simulink model "MSBR_Plant"  (R2021b)
settings: Solver=ode45  StartTime=0.0  StopTime=sim_time  MaxStep=ts_max  RelTol=1e-4
values from neighbouring files (symbols this model uses):
  a_1 = 8.7292e-2/wilson_ratio    (= 0.0087292)    [Whole_Plant_Cool_Pump_Accident_script.m]    (also in Whole_Plant_Fert_Pump_Accident_script.m; Whole_Plant_Fuel_Pump_Accident.m; Whole_Plant_Fuel_Pump_Accident_script.m; Whole_Plant_Reactivity_Accident.m)
  a_2 = 7.3787e-4/wilson_ratio    (= 7.3787e-05)    [Whole_Plant_Cool_Pump_Accident_script.m]    (also in Whole_Plant_Fert_Pump_Accident_script.m; Whole_Plant_Fuel_Pump_Accident.m; Whole_Plant_Fuel_Pump_Accident_script.m; Whole_Plant_Reactivity_Accident.m)
  a_b = 1.656e-5    (= 1.656e-05)    [Whole_Plant_Cool_Pump_Accident_script.m]    (also in Whole_Plant_Fert_Pump_Accident_script.m; Whole_Plant_Fuel_Pump_Accident.m; Whole_Plant_Fuel_Pump_Accident_script.m; Whole_Plant_Reactivity_Accident.m)
  a_f = -8.172e-5    (= -8.172e-05)    [Whole_Plant_Cool_Pump_Accident_script.m]    (also in Whole_Plant_Fert_Pump_Accident_script.m; Whole_Plant_Fuel_Pump_Accident.m; Whole_Plant_Fuel_Pump_Accident_script.m; Whole_Plant_Reactivity_Accident.m)
  a_g = 2.016e-5    (= 2.016e-05)    [Whole_Plant_Cool_Pump_Accident_script.m]    (also in Whole_Plant_Fert_Pump_Accident_script.m; Whole_Plant_Fuel_Pump_Accident.m; Whole_Plant_Fuel_Pump_Accident_script.m; Whole_Plant_Reactivity_Accident.m)
  A_s = pi()*((D_OTSG_i^2)/4) - A_w_OTSG - A_p_OTSG    [Whole_Plant_Cool_Pump_Accident_script.m]    (also in Whole_Plant_Fert_Pump_Accident_script.m; Whole_Plant_Fuel_Pump_Accident.m; Whole_Plant_Fuel_Pump_Accident_script.m; Whole_Plant_Reactivity_Accident.m)
  alpha_co = 316.2    [Whole_Plant_Cool_Pump_Accident_script.m]    (also in Whole_Plant_Fert_Pump_Accident_script.m; Whole_Plant_Fuel_Pump_Accident.m; Whole_Plant_Fuel_Pump_Accident_script.m; Whole_Plant_Reactivity_Accident.m)
  beta = [2.290e-04, 8.320e-04, 7.100e-04, 8.520e-04, 1.710e-04, 1.020e-04]    [Whole_Plant_Cool_Pump_Accident_script.m]    (also in Whole_Plant_Fert_Pump_Accident_script.m; Whole_Plant_Fuel_Pump_Accident.m; Whole_Plant_Fuel_Pump_Accident_script.m; Whole_Plant_Reactivity_Accident.m)
  beta_co = 68.0958    [Whole_Plant_Cool_Pump_Accident_script.m]    (also in Whole_Plant_Fert_Pump_Accident_script.m; Whole_Plant_Fuel_Pump_Accident.m; Whole_Plant_Fuel_Pump_Accident_script.m; Whole_Plant_Reactivity_Accident.m)
  beta_t = sum(beta)    [Whole_Plant_Cool_Pump_Accident_script.m]    (also in Whole_Plant_Fert_Pump_Accident_script.m; Whole_Plant_Fuel_Pump_Accident.m; Whole_Plant_Fuel_Pump_Accident_script.m; Whole_Plant_Reactivity_Accident.m)
  C_nc_X_A_nc = 12.8    [Whole_Plant_Cool_Pump_Accident_script.m]    (also in Whole_Plant_Fert_Pump_Accident_script.m; Whole_Plant_Fuel_Pump_Accident.m; Whole_Plant_Fuel_Pump_Accident_script.m; Whole_Plant_Reactivity_Accident.m)
  C_pcw = 0.0042    [Whole_Plant_Cool_Pump_Accident_script.m]    (also in Whole_Plant_Fert_Pump_Accident_script.m; Whole_Plant_Fuel_Pump_Accident.m; Whole_Plant_Fuel_Pump_Accident_script.m; Whole_Plant_Reactivity_Accident.m)
  C_rh_X_A_rh = 33    [Whole_Plant_Cool_Pump_Accident_script.m]    (also in Whole_Plant_Fert_Pump_Accident_script.m; Whole_Plant_Fuel_Pump_Accident.m; Whole_Plant_Fuel_Pump_Accident_script.m; Whole_Plant_Reactivity_Accident.m)
  C_v = 0.84    [Whole_Plant_Cool_Pump_Accident_script.m]    (also in Whole_Plant_Fert_Pump_Accident_script.m; Whole_Plant_Fuel_Pump_Accident.m; Whole_Plant_Fuel_Pump_Accident_script.m; Whole_Plant_Reactivity_Accident.m)
  ce1 = 1.2471e-07    [Whole_Plant_Cool_Pump_Accident_script.m]    (also in Whole_Plant_Fert_Pump_Accident_script.m; Whole_Plant_Fuel_Pump_Accident.m; Whole_Plant_Fuel_Pump_Accident_script.m; Whole_Plant_Reactivity_Accident.m)
  ce2 = 5.3816e-14    [Whole_Plant_Cool_Pump_Accident_script.m]    (also in Whole_Plant_Fert_Pump_Accident_script.m; Whole_Plant_Fuel_Pump_Accident.m; Whole_Plant_Fuel_Pump_Accident_script.m; Whole_Plant_Reactivity_Accident.m)
  ce3 = 3.3721e-08    [Whole_Plant_Cool_Pump_Accident_script.m]    (also in Whole_Plant_Fert_Pump_Accident_script.m; Whole_Plant_Fuel_Pump_Accident.m; Whole_Plant_Fuel_Pump_Accident_script.m; Whole_Plant_Reactivity_Accident.m)
  Cp_fw = XSteam('Cp_pT',P_set*10,T_fw)/1000    [Whole_Plant_Cool_Pump_Accident_script.m]    (also in Whole_Plant_Fert_Pump_Accident_script.m; Whole_Plant_Fuel_Pump_Accident.m; Whole_Plant_Fuel_Pump_Accident_script.m; Whole_Plant_Reactivity_Accident.m)
  Cp_p = Cp_sec    (= 0.001716588)    [Whole_Plant_Cool_Pump_Accident_script.m]    (also in Whole_Plant_Fert_Pump_Accident_script.m; Whole_Plant_Fuel_Pump_Accident.m; Whole_Plant_Fuel_Pump_Accident_script.m; Whole_Plant_Reactivity_Accident.m)
  Cp_rh = 0.0021520    (= 0.002152)    [Whole_Plant_Cool_Pump_Accident_script.m]    (also in Whole_Plant_Fert_Pump_Accident_script.m; Whole_Plant_Fuel_Pump_Accident.m; Whole_Plant_Fuel_Pump_Accident_script.m; Whole_Plant_Reactivity_Accident.m)
  Cp_s = XSteam('Cp_pT',P_s*10,T_s)/1000    [Whole_Plant_Cool_Pump_Accident_script.m]    (also in Whole_Plant_Fert_Pump_Accident_script.m; Whole_Plant_Fuel_Pump_Accident.m; Whole_Plant_Fuel_Pump_Accident_script.m; Whole_Plant_Reactivity_Accident.m)
  Cp_sc = XSteam('Cp_pT',P_set*10,T_sc2)/1000    [Whole_Plant_Cool_Pump_Accident_script.m]    (also in Whole_Plant_Fert_Pump_Accident_script.m; Whole_Plant_Fuel_Pump_Accident.m; Whole_Plant_Fuel_Pump_Accident_script.m; Whole_Plant_Reactivity_Accident.m)
  Cp_w = 468.992e-6    (= 0.000468992)    [Whole_Plant_Cool_Pump_Accident_script.m]    (also in Whole_Plant_Fert_Pump_Accident_script.m; Whole_Plant_Fuel_Pump_Accident.m; Whole_Plant_Fuel_Pump_Accident_script.m; Whole_Plant_Reactivity_Accident.m)
  D_it = D_ot-2*T_th    (= 0.014147)    [Whole_Plant_Cool_Pump_Accident_script.m]    (also in Whole_Plant_Fert_Pump_Accident_script.m; Whole_Plant_Fuel_Pump_Accident.m; Whole_Plant_Fuel_Pump_Accident_script.m; Whole_Plant_Reactivity_Accident.m)
  D_ot = 0.015875    [Whole_Plant_Cool_Pump_Accident_script.m]    (also in Whole_Plant_Fert_Pump_Accident_script.m; Whole_Plant_Fuel_Pump_Accident.m; Whole_Plant_Fuel_Pump_Accident_script.m; Whole_Plant_Reactivity_Accident.m)
  dHs_dPs = c(1)    [Whole_Plant_Cool_Pump_Accident_script.m]    (also in Whole_Plant_Fert_Pump_Accident_script.m; Whole_Plant_Fuel_Pump_Accident.m; Whole_Plant_Fuel_Pump_Accident_script.m; Whole_Plant_Reactivity_Accident.m)
  eta_hp_isen = 0.861    [Whole_Plant_Cool_Pump_Accident_script.m]    (also in Whole_Plant_Fert_Pump_Accident_script.m; Whole_Plant_Fuel_Pump_Accident.m; Whole_Plant_Fuel_Pump_Accident_script.m; Whole_Plant_Reactivity_Accident.m)
  eta_lp_isen = 0.861    [Whole_Plant_Cool_Pump_Accident_script.m]    (also in Whole_Plant_Fert_Pump_Accident_script.m; Whole_Plant_Fuel_Pump_Accident.m; Whole_Plant_Fuel_Pump_Accident_script.m; Whole_Plant_Reactivity_Accident.m)
  gamma_I = 5.1135e-2    (= 0.051135)    [Whole_Plant_Cool_Pump_Accident_script.m]    (also in Whole_Plant_Fert_Pump_Accident_script.m; Whole_Plant_Fuel_Pump_Accident.m; Whole_Plant_Fuel_Pump_Accident_script.m; Whole_Plant_Reactivity_Accident.m)
  gamma_Xe = 1.1628e-2    (= 0.011628)    [Whole_Plant_Cool_Pump_Accident_script.m]    (also in Whole_Plant_Fert_Pump_Accident_script.m; Whole_Plant_Fuel_Pump_Accident.m; Whole_Plant_Fuel_Pump_Accident_script.m; Whole_Plant_Reactivity_Accident.m)
  H_co0 = 0.149    [Whole_Plant_Cool_Pump_Accident_script.m]    (also in Whole_Plant_Fert_Pump_Accident_script.m; Whole_Plant_Fuel_Pump_Accident.m; Whole_Plant_Fuel_Pump_Accident_script.m; Whole_Plant_Reactivity_Accident.m)
  H_f_co0 = 0.149    [Whole_Plant_Cool_Pump_Accident_script.m]    (also in Whole_Plant_Fert_Pump_Accident_script.m; Whole_Plant_Fuel_Pump_Accident.m; Whole_Plant_Fuel_Pump_Accident_script.m; Whole_Plant_Reactivity_Accident.m)
  H_fg_co0 = 2.35    [Whole_Plant_Cool_Pump_Accident_script.m]    (also in Whole_Plant_Fert_Pump_Accident_script.m; Whole_Plant_Fuel_Pump_Accident.m; Whole_Plant_Fuel_Pump_Accident_script.m; Whole_Plant_Reactivity_Accident.m)
  H_fgrh0 = (XSteam('hV_p', P_s*1e1) - XSteam('hL_p', P_s*1e1))/1e3    [Whole_Plant_Cool_Pump_Accident_script.m]    (also in Whole_Plant_Fert_Pump_Accident_script.m; Whole_Plant_Fuel_Pump_Accident.m; Whole_Plant_Fuel_Pump_Accident_script.m; Whole_Plant_Reactivity_Accident.m)
  H_frh0 = XSteam('hL_p', P_s*1e1)/1e3    [Whole_Plant_Cool_Pump_Accident_script.m]    (also in Whole_Plant_Fert_Pump_Accident_script.m; Whole_Plant_Fuel_Pump_Accident.m; Whole_Plant_Fuel_Pump_Accident_script.m; Whole_Plant_Reactivity_Accident.m)
  h_fwh1 = 0.5927    [Whole_Plant_Cool_Pump_Accident_script.m]    (also in Whole_Plant_Fert_Pump_Accident_script.m; Whole_Plant_Fuel_Pump_Accident.m; Whole_Plant_Fuel_Pump_Accident_script.m; Whole_Plant_Reactivity_Accident.m)
  H_fwh10 = 0.46009    [Whole_Plant_Cool_Pump_Accident_script.m]    (also in Whole_Plant_Fert_Pump_Accident_script.m; Whole_Plant_Fuel_Pump_Accident.m; Whole_Plant_Fuel_Pump_Accident_script.m; Whole_Plant_Reactivity_Accident.m)
  h_fwh2 = 1.230803    [Whole_Plant_Cool_Pump_Accident_script.m]    (also in Whole_Plant_Fert_Pump_Accident_script.m; Whole_Plant_Fuel_Pump_Accident.m; Whole_Plant_Fuel_Pump_Accident_script.m; Whole_Plant_Reactivity_Accident.m)
  H_fwh20 = 0.6784    [Whole_Plant_Cool_Pump_Accident_script.m]    (also in Whole_Plant_Fert_Pump_Accident_script.m; Whole_Plant_Fuel_Pump_Accident.m; Whole_Plant_Fuel_Pump_Accident_script.m; Whole_Plant_Reactivity_Accident.m)
  H_grh0 = 2.8029    [Whole_Plant_Cool_Pump_Accident_script.m]    (also in Whole_Plant_Fert_Pump_Accident_script.m; Whole_Plant_Fuel_Pump_Accident.m; Whole_Plant_Fuel_Pump_Accident_script.m; Whole_Plant_Reactivity_Accident.m)
  H_hp_isen0 = 2.5111    [Whole_Plant_Cool_Pump_Accident_script.m]    (also in Whole_Plant_Fert_Pump_Accident_script.m; Whole_Plant_Fuel_Pump_Accident.m; Whole_Plant_Fuel_Pump_Accident_script.m; Whole_Plant_Reactivity_Accident.m)
  H_hpt_out = 2.6201    [Whole_Plant_Cool_Pump_Accident_script.m]    (also in Whole_Plant_Fert_Pump_Accident_script.m; Whole_Plant_Fuel_Pump_Accident.m; Whole_Plant_Fuel_Pump_Accident_script.m; Whole_Plant_Reactivity_Accident.m)
  H_lp_isen = 958.4*1054.35e-6/0.45359237    (= 2.22774699671)    [Whole_Plant_Cool_Pump_Accident_script.m]    (also in Whole_Plant_Fert_Pump_Accident_script.m; Whole_Plant_Fuel_Pump_Accident.m; Whole_Plant_Fuel_Pump_Accident_script.m; Whole_Plant_Reactivity_Accident.m)
  H_lpt_out = 2.3089    [Whole_Plant_Cool_Pump_Accident_script.m]    (also in Whole_Plant_Fert_Pump_Accident_script.m; Whole_Plant_Fuel_Pump_Accident.m; Whole_Plant_Fuel_Pump_Accident_script.m; Whole_Plant_Reactivity_Accident.m)
  H_nc = XSteam('h_pT', P_s*10, T_s)/1000    [Whole_Plant_Cool_Pump_Accident_script.m]    (also in Whole_Plant_Fert_Pump_Accident_script.m; Whole_Plant_Fuel_Pump_Accident.m; Whole_Plant_Fuel_Pump_Accident_script.m; Whole_Plant_Reactivity_Accident.m)
  h_pw = h_s    (= 0.02555)    [Whole_Plant_Cool_Pump_Accident_script.m]    (also in Whole_Plant_Fert_Pump_Accident_script.m; Whole_Plant_Fuel_Pump_Accident.m; Whole_Plant_Fuel_Pump_Accident_script.m; Whole_Plant_Reactivity_Accident.m)
  H_rh = 2.8115    [Whole_Plant_Cool_Pump_Accident_script.m]    (also in Whole_Plant_Fert_Pump_Accident_script.m; Whole_Plant_Fuel_Pump_Accident.m; Whole_Plant_Fuel_Pump_Accident_script.m; Whole_Plant_Reactivity_Accident.m)
  h_wb = 13349.334646671E-6    (= 0.0133493346467)    [Whole_Plant_Cool_Pump_Accident_script.m]    (also in Whole_Plant_Fert_Pump_Accident_script.m; Whole_Plant_Fuel_Pump_Accident.m; Whole_Plant_Fuel_Pump_Accident_script.m; Whole_Plant_Reactivity_Accident.m)
  h_ws = 5732.378387768E-6    (= 0.00573237838777)    [Whole_Plant_Cool_Pump_Accident_script.m]    (also in Whole_Plant_Fert_Pump_Accident_script.m; Whole_Plant_Fuel_Pump_Accident.m; Whole_Plant_Fuel_Pump_Accident_script.m; Whole_Plant_Reactivity_Accident.m)
  h_wsc = 8385.005556375E-6    (= 0.00838500555638)    [Whole_Plant_Cool_Pump_Accident_script.m]    (also in Whole_Plant_Fert_Pump_Accident_script.m; Whole_Plant_Fuel_Pump_Accident.m; Whole_Plant_Fuel_Pump_Accident_script.m; Whole_Plant_Reactivity_Accident.m)
  hA_bg = A_fert*h_bg    (= 2.76411813627)    [Whole_Plant_Cool_Pump_Accident_script.m]    (also in Whole_Plant_Fert_Pump_Accident_script.m; Whole_Plant_Fuel_Pump_Accident.m; Whole_Plant_Fuel_Pump_Accident_script.m; Whole_Plant_Reactivity_Accident.m)
  hA_co0 = 140    [Whole_Plant_Cool_Pump_Accident_script.m]    (also in Whole_Plant_Fert_Pump_Accident_script.m; Whole_Plant_Fuel_Pump_Accident.m; Whole_Plant_Fuel_Pump_Accident_script.m; Whole_Plant_Reactivity_Accident.m)
  hA_fg_dn = h_fg*A_fuel_down    [Whole_Plant_Cool_Pump_Accident_script.m]    (also in Whole_Plant_Fert_Pump_Accident_script.m; Whole_Plant_Fuel_Pump_Accident.m; Whole_Plant_Fuel_Pump_Accident_script.m; Whole_Plant_Reactivity_Accident.m)
  hA_fg_up = h_fg*A_fuel_up    [Whole_Plant_Cool_Pump_Accident_script.m]    (also in Whole_Plant_Fert_Pump_Accident_script.m; Whole_Plant_Fuel_Pump_Accident.m; Whole_Plant_Fuel_Pump_Accident_script.m; Whole_Plant_Reactivity_Accident.m)
  hA_p_bhx1 = [h_pb*A_pbhx/2,h_pb*A_pbhx/2]    [Whole_Plant_Cool_Pump_Accident_script.m]    (also in Whole_Plant_Fert_Pump_Accident_script.m; Whole_Plant_Fuel_Pump_Accident.m; Whole_Plant_Fuel_Pump_Accident_script.m; Whole_Plant_Reactivity_Accident.m)
  hA_p_bhx2 = hA_p_bhx1    [Whole_Plant_Cool_Pump_Accident_script.m]    (also in Whole_Plant_Fert_Pump_Accident_script.m; Whole_Plant_Fuel_Pump_Accident.m; Whole_Plant_Fuel_Pump_Accident_script.m; Whole_Plant_Reactivity_Accident.m)
  hA_p_bhx3 = hA_p_bhx1    [Whole_Plant_Cool_Pump_Accident_script.m]    (also in Whole_Plant_Fert_Pump_Accident_script.m; Whole_Plant_Fuel_Pump_Accident.m; Whole_Plant_Fuel_Pump_Accident_script.m; Whole_Plant_Reactivity_Accident.m)
  hA_p_bhx4 = hA_p_bhx1    [Whole_Plant_Cool_Pump_Accident_script.m]    (also in Whole_Plant_Fert_Pump_Accident_script.m; Whole_Plant_Fuel_Pump_Accident.m; Whole_Plant_Fuel_Pump_Accident_script.m; Whole_Plant_Reactivity_Accident.m)
  hA_p_fhx1 = [h_p*A_pfhx_dn/2,h_p*A_pfhx_dn/2,h_p*A_pfhx_up/2,h_p*A_pfhx_up/2]    [Whole_Plant_Cool_Pump_Accident_script.m]    (also in Whole_Plant_Fert_Pump_Accident_script.m; Whole_Plant_Fuel_Pump_Accident.m; Whole_Plant_Fuel_Pump_Accident_script.m; Whole_Plant_Reactivity_Accident.m)
  hA_p_fhx2 = hA_p_fhx1    [Whole_Plant_Cool_Pump_Accident_script.m]    (also in Whole_Plant_Fert_Pump_Accident_script.m; Whole_Plant_Fuel_Pump_Accident.m; Whole_Plant_Fuel_Pump_Accident_script.m; Whole_Plant_Reactivity_Accident.m)
  hA_p_fhx3 = hA_p_fhx1    [Whole_Plant_Cool_Pump_Accident_script.m]    (also in Whole_Plant_Fert_Pump_Accident_script.m; Whole_Plant_Fuel_Pump_Accident.m; Whole_Plant_Fuel_Pump_Accident_script.m; Whole_Plant_Reactivity_Accident.m)
  hA_p_fhx4 = hA_p_fhx1    [Whole_Plant_Cool_Pump_Accident_script.m]    (also in Whole_Plant_Fert_Pump_Accident_script.m; Whole_Plant_Fuel_Pump_Accident.m; Whole_Plant_Fuel_Pump_Accident_script.m; Whole_Plant_Reactivity_Accident.m)
  hA_s_bhx1 = [h_sb*A_sbhx/2,h_sb*A_sbhx/2]    [Whole_Plant_Cool_Pump_Accident_script.m]    (also in Whole_Plant_Fert_Pump_Accident_script.m; Whole_Plant_Fuel_Pump_Accident.m; Whole_Plant_Fuel_Pump_Accident_script.m; Whole_Plant_Reactivity_Accident.m)
  hA_s_bhx2 = hA_s_bhx1    [Whole_Plant_Cool_Pump_Accident_script.m]    (also in Whole_Plant_Fert_Pump_Accident_script.m; Whole_Plant_Fuel_Pump_Accident.m; Whole_Plant_Fuel_Pump_Accident_script.m; Whole_Plant_Reactivity_Accident.m)
  hA_s_bhx3 = hA_s_bhx1    [Whole_Plant_Cool_Pump_Accident_script.m]    (also in Whole_Plant_Fert_Pump_Accident_script.m; Whole_Plant_Fuel_Pump_Accident.m; Whole_Plant_Fuel_Pump_Accident_script.m; Whole_Plant_Reactivity_Accident.m)
  hA_s_bhx4 = hA_s_bhx1    [Whole_Plant_Cool_Pump_Accident_script.m]    (also in Whole_Plant_Fert_Pump_Accident_script.m; Whole_Plant_Fuel_Pump_Accident.m; Whole_Plant_Fuel_Pump_Accident_script.m; Whole_Plant_Reactivity_Accident.m)
  hA_s_fhx1 = [h_s*A_sfhx_up/2,h_s*A_sfhx_up/2,h_s*A_sfhx_dn/2,h_s*A_sfhx_dn/2]    [Whole_Plant_Cool_Pump_Accident_script.m]    (also in Whole_Plant_Fert_Pump_Accident_script.m; Whole_Plant_Fuel_Pump_Accident.m; Whole_Plant_Fuel_Pump_Accident_script.m; Whole_Plant_Reactivity_Accident.m)
  hA_s_fhx2 = hA_s_fhx1    [Whole_Plant_Cool_Pump_Accident_script.m]    (also in Whole_Plant_Fert_Pump_Accident_script.m; Whole_Plant_Fuel_Pump_Accident.m; Whole_Plant_Fuel_Pump_Accident_script.m; Whole_Plant_Reactivity_Accident.m)
  hA_s_fhx3 = hA_s_fhx1    [Whole_Plant_Cool_Pump_Accident_script.m]    (also in Whole_Plant_Fert_Pump_Accident_script.m; Whole_Plant_Fuel_Pump_Accident.m; Whole_Plant_Fuel_Pump_Accident_script.m; Whole_Plant_Reactivity_Accident.m)
  hA_s_fhx4 = hA_s_fhx1    [Whole_Plant_Cool_Pump_Accident_script.m]    (also in Whole_Plant_Fert_Pump_Accident_script.m; Whole_Plant_Fuel_Pump_Accident.m; Whole_Plant_Fuel_Pump_Accident_script.m; Whole_Plant_Reactivity_Accident.m)
  I_0 = gamma_I*Sigma_f_msbr*phi_0/lam_I    (= 1.30000734126e+17)    [Whole_Plant_Cool_Pump_Accident_script.m]    (also in Whole_Plant_Fert_Pump_Accident_script.m; Whole_Plant_Fuel_Pump_Accident.m; Whole_Plant_Fuel_Pump_Accident_script.m; Whole_Plant_Reactivity_Accident.m)
  k_1 = 0.5    [Whole_Plant_Cool_Pump_Accident_script.m]    (also in Whole_Plant_Fert_Pump_Accident_script.m; Whole_Plant_Fuel_Pump_Accident.m; Whole_Plant_Fuel_Pump_Accident_script.m; Whole_Plant_Reactivity_Accident.m)
  K_1 = e(1)    [Whole_Plant_Cool_Pump_Accident_script.m]    (also in Whole_Plant_Fert_Pump_Accident_script.m; Whole_Plant_Fuel_Pump_Accident.m; Whole_Plant_Fuel_Pump_Accident_script.m; Whole_Plant_Reactivity_Accident.m)
  k_1b = 0.5    [Whole_Plant_Cool_Pump_Accident_script.m]    (also in Whole_Plant_Fert_Pump_Accident_script.m; Whole_Plant_Fuel_Pump_Accident.m; Whole_Plant_Fuel_Pump_Accident_script.m; Whole_Plant_Reactivity_Accident.m)
  k_2 = 0.5    [Whole_Plant_Cool_Pump_Accident_script.m]    (also in Whole_Plant_Fert_Pump_Accident_script.m; Whole_Plant_Fuel_Pump_Accident.m; Whole_Plant_Fuel_Pump_Accident_script.m; Whole_Plant_Reactivity_Accident.m)
  k_2b = 0.5    [Whole_Plant_Cool_Pump_Accident_script.m]    (also in Whole_Plant_Fert_Pump_Accident_script.m; Whole_Plant_Fuel_Pump_Accident.m; Whole_Plant_Fuel_Pump_Accident_script.m; Whole_Plant_Reactivity_Accident.m)
  k_3 = 0.5    [Whole_Plant_Cool_Pump_Accident_script.m]    (also in Whole_Plant_Fert_Pump_Accident_script.m; Whole_Plant_Fuel_Pump_Accident.m; Whole_Plant_Fuel_Pump_Accident_script.m; Whole_Plant_Reactivity_Accident.m)
  k_4 = 0.5    [Whole_Plant_Cool_Pump_Accident_script.m]    (also in Whole_Plant_Fert_Pump_Accident_script.m; Whole_Plant_Fuel_Pump_Accident.m; Whole_Plant_Fuel_Pump_Accident_script.m; Whole_Plant_Reactivity_Accident.m)
  K_4 = b(1)    [Whole_Plant_Cool_Pump_Accident_script.m]    (also in Whole_Plant_Fert_Pump_Accident_script.m; Whole_Plant_Fuel_Pump_Accident.m; Whole_Plant_Fuel_Pump_Accident_script.m; Whole_Plant_Reactivity_Accident.m)
  K_5 = a(1)    [Whole_Plant_Cool_Pump_Accident_script.m]    (also in Whole_Plant_Fert_Pump_Accident_script.m; Whole_Plant_Fuel_Pump_Accident.m; Whole_Plant_Fuel_Pump_Accident_script.m; Whole_Plant_Reactivity_Accident.m)
  K_b = d(1)    [Whole_Plant_Cool_Pump_Accident_script.m]    (also in Whole_Plant_Fert_Pump_Accident_script.m; Whole_Plant_Fuel_Pump_Accident.m; Whole_Plant_Fuel_Pump_Accident_script.m; Whole_Plant_Reactivity_Accident.m)
  k_b1 = (K_B/2)/K    (= 0.0089463103122)    [Whole_Plant_Cool_Pump_Accident_script.m]    (also in Whole_Plant_Fert_Pump_Accident_script.m; Whole_Plant_Fuel_Pump_Accident.m; Whole_Plant_Fuel_Pump_Accident_script.m; Whole_Plant_Reactivity_Accident.m)
  k_b2 = k_b1    (= 0.0089463103122)    [Whole_Plant_Cool_Pump_Accident_script.m]    (also in Whole_Plant_Fert_Pump_Accident_script.m; Whole_Plant_Fuel_Pump_Accident.m; Whole_Plant_Fuel_Pump_Accident_script.m; Whole_Plant_Reactivity_Accident.m)
  K_bhp = 0.1634    [Whole_Plant_Cool_Pump_Accident_script.m]    (also in Whole_Plant_Fert_Pump_Accident_script.m; Whole_Plant_Fuel_Pump_Accident.m; Whole_Plant_Fuel_Pump_Accident_script.m; Whole_Plant_Reactivity_Accident.m)
  K_blp = 0.2174    [Whole_Plant_Cool_Pump_Accident_script.m]    (also in Whole_Plant_Fert_Pump_Accident_script.m; Whole_Plant_Fuel_Pump_Accident.m; Whole_Plant_Fuel_Pump_Accident_script.m; Whole_Plant_Reactivity_Accident.m)
  k_f1 = ((1 - K_G - K_B - K_Ba)/4)/K    (= 0.226055463576)    [Whole_Plant_Cool_Pump_Accident_script.m]    (also in Whole_Plant_Fert_Pump_Accident_script.m; Whole_Plant_Fuel_Pump_Accident.m; Whole_Plant_Fuel_Pump_Accident_script.m; Whole_Plant_Reactivity_Accident.m)
  k_f2 = k_f1    (= 0.226055463576)    [Whole_Plant_Cool_Pump_Accident_script.m]    (also in Whole_Plant_Fert_Pump_Accident_script.m; Whole_Plant_Fuel_Pump_Accident.m; Whole_Plant_Fuel_Pump_Accident_script.m; Whole_Plant_Reactivity_Accident.m)
  k_f3 = k_f1    (= 0.226055463576)    [Whole_Plant_Cool_Pump_Accident_script.m]    (also in Whole_Plant_Fert_Pump_Accident_script.m; Whole_Plant_Fuel_Pump_Accident.m; Whole_Plant_Fuel_Pump_Accident_script.m; Whole_Plant_Reactivity_Accident.m)
  k_f4 = k_f1    (= 0.226055463576)    [Whole_Plant_Cool_Pump_Accident_script.m]    (also in Whole_Plant_Fert_Pump_Accident_script.m; Whole_Plant_Fuel_Pump_Accident.m; Whole_Plant_Fuel_Pump_Accident_script.m; Whole_Plant_Reactivity_Accident.m)
  k_g1 = ((K_G*K_fuel)/2)/K    (= 0.0346590586566)    [Whole_Plant_Cool_Pump_Accident_script.m]    (also in Whole_Plant_Fert_Pump_Accident_script.m; Whole_Plant_Fuel_Pump_Accident.m; Whole_Plant_Fuel_Pump_Accident_script.m; Whole_Plant_Reactivity_Accident.m)
  k_g2 = k_g1    (= 0.0346590586566)    [Whole_Plant_Cool_Pump_Accident_script.m]    (also in Whole_Plant_Fert_Pump_Accident_script.m; Whole_Plant_Fuel_Pump_Accident.m; Whole_Plant_Fuel_Pump_Accident_script.m; Whole_Plant_Reactivity_Accident.m)
  k_g3 = (K_G*(1-K_fuel))/K    (= 0.00856740775781)    [Whole_Plant_Cool_Pump_Accident_script.m]    (also in Whole_Plant_Fert_Pump_Accident_script.m; Whole_Plant_Fuel_Pump_Accident.m; Whole_Plant_Fuel_Pump_Accident_script.m; Whole_Plant_Reactivity_Accident.m)
  K_sc = f(1)    [Whole_Plant_Cool_Pump_Accident_script.m]    (also in Whole_Plant_Fert_Pump_Accident_script.m; Whole_Plant_Fuel_Pump_Accident.m; Whole_Plant_Fuel_Pump_Accident_script.m; Whole_Plant_Reactivity_Accident.m)
  L = 22.0    (= 22)    [Whole_Plant_Cool_Pump_Accident_script.m]    (also in Whole_Plant_Fert_Pump_Accident_script.m; Whole_Plant_Fuel_Pump_Accident.m; Whole_Plant_Fuel_Pump_Accident_script.m; Whole_Plant_Reactivity_Accident.m)
  L_b = 1.9    [Whole_Plant_Cool_Pump_Accident_script.m]    (also in Whole_Plant_Fert_Pump_Accident_script.m; Whole_Plant_Fuel_Pump_Accident.m; Whole_Plant_Fuel_Pump_Accident_script.m; Whole_Plant_Reactivity_Accident.m)
  L_s = 16.53    [Whole_Plant_Cool_Pump_Accident_script.m]    (also in Whole_Plant_Fert_Pump_Accident_script.m; Whole_Plant_Fuel_Pump_Accident.m; Whole_Plant_Fuel_Pump_Accident_script.m; Whole_Plant_Reactivity_Accident.m)
  L_sc = L-L_b-L_s    (= 3.57)    [Whole_Plant_Cool_Pump_Accident_script.m]    (also in Whole_Plant_Fert_Pump_Accident_script.m; Whole_Plant_Fuel_Pump_Accident.m; Whole_Plant_Fuel_Pump_Accident_script.m; Whole_Plant_Reactivity_Accident.m)
  Lam = 3.3e-4    (= 0.00033)    [Whole_Plant_Cool_Pump_Accident_script.m]    (also in Whole_Plant_Fert_Pump_Accident_script.m; Whole_Plant_Fuel_Pump_Accident.m; Whole_Plant_Fuel_Pump_Accident_script.m; Whole_Plant_Reactivity_Accident.m)
  lam = [1.260e-02, 3.370e-02, 1.390e-01, 3.250e-01, 1.130e+00, 2.500e+00]    [Whole_Plant_Cool_Pump_Accident_script.m]    (also in Whole_Plant_Fert_Pump_Accident_script.m; Whole_Plant_Fuel_Pump_Accident.m; Whole_Plant_Fuel_Pump_Accident_script.m; Whole_Plant_Reactivity_Accident.m)
  lam_bubl = 2.0e-2    (= 0.02)    [Whole_Plant_Cool_Pump_Accident_script.m]    (also in Whole_Plant_Fert_Pump_Accident_script.m; Whole_Plant_Fuel_Pump_Accident.m; Whole_Plant_Fuel_Pump_Accident_script.m; Whole_Plant_Reactivity_Accident.m)
  lam_I = 2.875e-5    (= 2.875e-05)    [Whole_Plant_Cool_Pump_Accident_script.m]    (also in Whole_Plant_Fert_Pump_Accident_script.m; Whole_Plant_Fuel_Pump_Accident.m; Whole_Plant_Fuel_Pump_Accident_script.m; Whole_Plant_Reactivity_Accident.m)
  lam_Xe = 2.0916e-5    (= 2.0916e-05)    [Whole_Plant_Cool_Pump_Accident_script.m]    (also in Whole_Plant_Fert_Pump_Accident_script.m; Whole_Plant_Fuel_Pump_Accident.m; Whole_Plant_Fuel_Pump_Accident_script.m; Whole_Plant_Reactivity_Accident.m)
  m_bm = (W_b1+W_b2+W_b3+W_b4)*time_mixb    (= 2167.1636)    [Whole_Plant_Cool_Pump_Accident_script.m]    (also in Whole_Plant_Fert_Pump_Accident_script.m; Whole_Plant_Fuel_Pump_Accident.m; Whole_Plant_Fuel_Pump_Accident_script.m; Whole_Plant_Reactivity_Accident.m)
  M_cw = 65000    [Whole_Plant_Cool_Pump_Accident_script.m]    (also in Whole_Plant_Fert_Pump_Accident_script.m; Whole_Plant_Fuel_Pump_Accident.m; Whole_Plant_Fuel_Pump_Accident_script.m; Whole_Plant_Reactivity_Accident.m)
  m_fm = (W_f1+W_f2+W_f3+W_f4)*time_mixf    (= 5443.108)    [Whole_Plant_Cool_Pump_Accident_script.m]    (also in Whole_Plant_Fert_Pump_Accident_script.m; Whole_Plant_Fuel_Pump_Accident.m; Whole_Plant_Fuel_Pump_Accident_script.m; Whole_Plant_Reactivity_Accident.m)
  M_hw0 = 10000    [Whole_Plant_Cool_Pump_Accident_script.m]    (also in Whole_Plant_Fert_Pump_Accident_script.m; Whole_Plant_Fuel_Pump_Accident.m; Whole_Plant_Fuel_Pump_Accident_script.m; Whole_Plant_Reactivity_Accident.m)
  m_sm = (W_s1+W_s2+W_s3+W_s4)*time_mixs    (= 8467.056)    [Whole_Plant_Cool_Pump_Accident_script.m]    (also in Whole_Plant_Fert_Pump_Accident_script.m; Whole_Plant_Fuel_Pump_Accident.m; Whole_Plant_Fuel_Pump_Accident_script.m; Whole_Plant_Reactivity_Accident.m)
  M_stm = 0.018    [Whole_Plant_Cool_Pump_Accident_script.m]    (also in Whole_Plant_Fert_Pump_Accident_script.m; Whole_Plant_Fuel_Pump_Accident.m; Whole_Plant_Fuel_Pump_Accident_script.m; Whole_Plant_Reactivity_Accident.m)
  mcp_b1 = mass_bn*Cp_b    (= 4.17494922705)    [Whole_Plant_Cool_Pump_Accident_script.m]    (also in Whole_Plant_Fert_Pump_Accident_script.m; Whole_Plant_Fuel_Pump_Accident.m; Whole_Plant_Fuel_Pump_Accident_script.m; Whole_Plant_Reactivity_Accident.m)
  mcp_b2 = mcp_b1    (= 4.17494922705)    [Whole_Plant_Cool_Pump_Accident_script.m]    (also in Whole_Plant_Fert_Pump_Accident_script.m; Whole_Plant_Fuel_Pump_Accident.m; Whole_Plant_Fuel_Pump_Accident_script.m; Whole_Plant_Reactivity_Accident.m)
  mcp_f1 = mass_fn*Cp_f    (= 5.5019469141)    [Whole_Plant_Cool_Pump_Accident_script.m]    (also in Whole_Plant_Fert_Pump_Accident_script.m; Whole_Plant_Fuel_Pump_Accident.m; Whole_Plant_Fuel_Pump_Accident_script.m; Whole_Plant_Reactivity_Accident.m)
  mcp_f2 = mass_fn*Cp_f    (= 5.5019469141)    [Whole_Plant_Cool_Pump_Accident_script.m]    (also in Whole_Plant_Fert_Pump_Accident_script.m; Whole_Plant_Fuel_Pump_Accident.m; Whole_Plant_Fuel_Pump_Accident_script.m; Whole_Plant_Reactivity_Accident.m)
  mcp_f3 = mass_fn*Cp_f    (= 5.5019469141)    [Whole_Plant_Cool_Pump_Accident_script.m]    (also in Whole_Plant_Fert_Pump_Accident_script.m; Whole_Plant_Fuel_Pump_Accident.m; Whole_Plant_Fuel_Pump_Accident_script.m; Whole_Plant_Reactivity_Accident.m)
  mcp_f4 = mass_fn*Cp_f    (= 5.5019469141)    [Whole_Plant_Cool_Pump_Accident_script.m]    (also in Whole_Plant_Fert_Pump_Accident_script.m; Whole_Plant_Fuel_Pump_Accident.m; Whole_Plant_Fuel_Pump_Accident_script.m; Whole_Plant_Reactivity_Accident.m)
  mcp_g1 = (mass_grap*Cp_g)*K_fuel/2    (= 32.9814988203)    [Whole_Plant_Cool_Pump_Accident_script.m]    (also in Whole_Plant_Fert_Pump_Accident_script.m; Whole_Plant_Fuel_Pump_Accident.m; Whole_Plant_Fuel_Pump_Accident_script.m; Whole_Plant_Reactivity_Accident.m)
  mcp_g2 = mcp_g1    (= 32.9814988203)    [Whole_Plant_Cool_Pump_Accident_script.m]    (also in Whole_Plant_Fert_Pump_Accident_script.m; Whole_Plant_Fuel_Pump_Accident.m; Whole_Plant_Fuel_Pump_Accident_script.m; Whole_Plant_Reactivity_Accident.m)
  mcp_g3 = (mass_grap*Cp_g)*(1-K_fuel)    (= 8.15273004546)    [Whole_Plant_Cool_Pump_Accident_script.m]    (also in Whole_Plant_Fert_Pump_Accident_script.m; Whole_Plant_Fuel_Pump_Accident.m; Whole_Plant_Fuel_Pump_Accident_script.m; Whole_Plant_Reactivity_Accident.m)
  mcp_p_bhx1 = mp_bhx1*Cp_b    [Whole_Plant_Cool_Pump_Accident_script.m]    (also in Whole_Plant_Fert_Pump_Accident_script.m; Whole_Plant_Fuel_Pump_Accident.m; Whole_Plant_Fuel_Pump_Accident_script.m; Whole_Plant_Reactivity_Accident.m)
  mcp_p_bhx2 = mp_bhx2*Cp_b    [Whole_Plant_Cool_Pump_Accident_script.m]    (also in Whole_Plant_Fert_Pump_Accident_script.m; Whole_Plant_Fuel_Pump_Accident.m; Whole_Plant_Fuel_Pump_Accident_script.m; Whole_Plant_Reactivity_Accident.m)
  mcp_p_bhx3 = mp_bhx3*Cp_b    [Whole_Plant_Cool_Pump_Accident_script.m]    (also in Whole_Plant_Fert_Pump_Accident_script.m; Whole_Plant_Fuel_Pump_Accident.m; Whole_Plant_Fuel_Pump_Accident_script.m; Whole_Plant_Reactivity_Accident.m)
  ... (+213 more)
undefined symbols (not defined in the file or in its folder): C0, H_con_table, H_convap_table, H_rh_table, H_rh_table1, H_rh_table2, H_rhvap_table, H_s_table, H_table, P_con_table, P_nc_table, P_rh_table, P_rh_table1, pres_table, rho_rh_table, rho_table, SV_nc_table, SVf_nc_table, temp_table
(part 1 of 13)
settings Model: Creator=Stephen Chase Pair  LastModifiedBy=Stephen Chase Pair
settings DataIOCC: ReturnWorkspaceOutputs=off

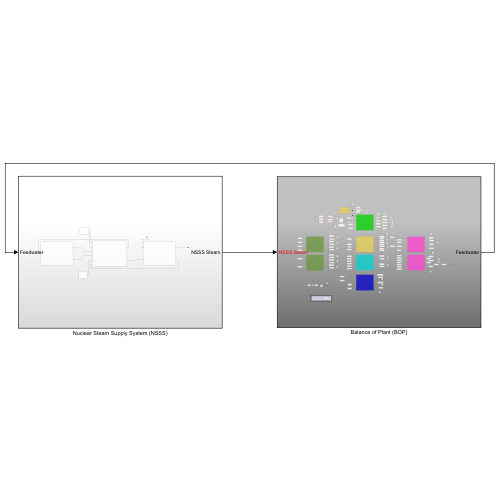
[thumbnail: Simulink's stored preview of the top-level diagram]
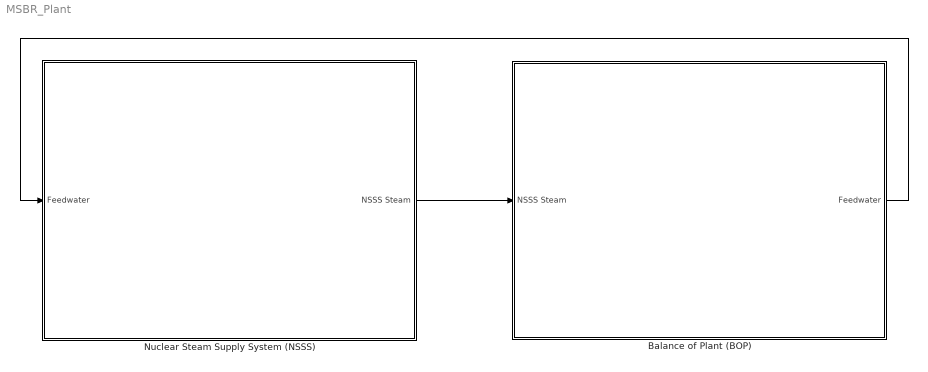
== system MSBR_Plant ==
  Balance of Plant (BOP) : Subsystem
  Nuclear Steam Supply System (NSSS) : Subsystem
  wires:
  Nuclear Steam Supply System (NSSS)/1(NSSS Steam) -> Balance of Plant (BOP)/1(NSSS Steam)
  Balance of Plant (BOP)/1(Feedwater) -> Nuclear Steam Supply System (NSSS)/1(Feedwater)

== system MSBR_Plant/Balance of Plant (BOP) ==
  note: 2-D lookup table returns steam enthalpy in MJ/kg for inputs i. Temperature in C, ii. Pressure in Pa
  In Bus Element : Inport  PortName=NSSS Steam  Element=Steam Temperature
  In Bus Element1 : Inport  PortName=NSSS Steam  Element=Steam Pressure
  In Bus Element2 : Inport  PortName=NSSS Steam  Element=Steam Flow Rate
  CONDENSER : Subsystem
  Constant19 : Constant  Value=482.63
  Display{6..11,13,26..46} (28 alike) : Display
  FEEDWATER HEATER 1 - LOW-PRESSURE : Subsystem
  FEEDWATER HEATER 2 - HIGH-PRESSURE : Subsystem
  Flow of Cooling Water Input : Constant  Value=W_cwi
  HIGH PRESSURE TURBINE : Subsystem
  LOW PRESSURE TURBINE : Subsystem
  MOISTURE SEPARATOR : Subsystem
  NOZZLE CHEST : Subsystem
  REHEATER : Subsystem
  Scope{,1..2,4..32} (32 alike) : Scope
  Secondary Steam Valve : Subsystem
  Steam Enthalpy : Lookup_n-D  BreakpointsForDimension1=temp_table  BreakpointsForDimension2=pres_table  Table=H_s_table  DiagnosticForOutOfRangeInput=Warning  InternalRulePriority=Speed  RndMeth=Simplest  InputSameDT=on
      settings: InputPortMap=u0,u1
  Sum : Sum  Inputs=-+|
  Temperature of Cooling Water Input : Constant  Value=T_cwi
  Out Bus Element : Outport  PortName=Feedwater  Element=Feedwater Temp
  Out Bus Element1 : Outport  PortName=Feedwater  Element=Feedwater Flow
  wires:
  NOZZLE CHEST/1(Enthalpy of Vaporization) -> Scope6/1, [H_fg_nc], Display6/1
  [H_hp] -> NOZZLE CHEST/3(Steam Enthalpy HP Turbine)
  NOZZLE CHEST/4(Steam Enthalpy in Nozzle Chest) -> Scope10/1, [H_nc], Display9/1
  NOZZLE CHEST/3(Steam Flow Rate in Nozzle Chest) -> Scope9/1, [steam_flow_nc], Display8/1
  [P_steam_OTSG] -> Scope30/1, Steam Enthalpy/2
  Sum/1 -> Display26/1, Scope5/1, NOZZLE CHEST/1(Steam Flow Rate OTSG)
  Steam Enthalpy/1 -> Scope/1, NOZZLE CHEST/2(Steam Enthalpy OTSG), Display13/1
  NOZZLE CHEST/5(Steam Pressure in Nozzle Chest) -> Scope11/1, [P_steam_nc], Display10/1
  [steam_flow_OTSG] -> Scope32/1, Secondary Steam Valve/1(Steam from OTSG), Sum/2
  [P_steam_rh] -> NOZZLE CHEST/4(Steam Pressure Reheater)
  Secondary Steam Valve/1(Steam to Reheater) -> Scope4/1, Display11/1, [steam_flow_reheat], Sum/1
  [flow_rh_lpt] -> LOW PRESSURE TURBINE/1(Flow from Reheater)
  [H_fg_nc] -> MOISTURE SEPARATOR/1(Enthalpy of Vaporization)
  LOW PRESSURE TURBINE/2(Steam Bleed Flow Rate LP Turbine) -> Scope22/1, [steam_bleed_lp], Display37/1
  FEEDWATER HEATER 2 - HIGH-PRESSURE/3(Feedwater Flow Rate) -> Scope28/1, [flow_fwh2_OTSG], Display45/1
  REHEATER/2(Flow to Feedwater Heater 2) -> Scope16/1, [flow_rh_fwh2], Display33/1
  MOISTURE SEPARATOR/1(Flow to Heater 2) -> Scope24/1, [flow_ms_fwh2], Display30/1
  REHEATER/3(Steam Pressure Reheater) -> Scope17/1, [P_steam_rh], Display34/1
  MOISTURE SEPARATOR/2(Flow to Reheater) -> Scope25/1, [flow_ms_rh], Display31/1
  [flow_rh_fwh2] -> FEEDWATER HEATER 2 - HIGH-PRESSURE/3(Flow from Reheater)
  [H_fwh1] -> FEEDWATER HEATER 2 - HIGH-PRESSURE/6(Enthalpy of Feedwater Heater 1)
  [flow_ms_rh] -> FEEDWATER HEATER 2 - HIGH-PRESSURE/4("Flow from Moisture Seperator to Reheater ")
  [P_steam_nc] -> HIGH PRESSURE TURBINE/3(Steam Pressure Nozzle Chest)
  [P_steam_rh] -> HIGH PRESSURE TURBINE/4(Steam Pressure Reheater)
  [H_nc] -> HIGH PRESSURE TURBINE/2(Steam Enthalpy Nozzle Chest)
  LOW PRESSURE TURBINE/3(Steam Enthalpy LP Turbine) -> Display42/1, Scope23/1, [H_lp]
  LOW PRESSURE TURBINE/1(Steam Flow Rate LP Turbine) -> Scope21/1, [steam_flow_lp], Display36/1
  [steam_bleed_lp] -> FEEDWATER HEATER 1 - LOW-PRESSURE/2(Steam Bleed Flow Rate LP Turbine)
  [flow_ms_fwh2] -> FEEDWATER HEATER 2 - HIGH-PRESSURE/2(Flow from Moisture Seperator)
  [flow_fwh2_fwh1] -> FEEDWATER HEATER 1 - LOW-PRESSURE/3(Flow from Feedwater Heater 2)
  [flow_fwh1_fwh2] -> FEEDWATER HEATER 2 - HIGH-PRESSURE/5(Flow from Feedwater Heater 1)
  [H_lp] -> CONDENSER/2(Steam Enthalpy LP Turbine)
  FEEDWATER HEATER 1 - LOW-PRESSURE/2(Feedwater Flow Rate) -> Scope20/1, Display39/1, [flow_fwh1_fwh2]
  [H_rh_nc] -> MOISTURE SEPARATOR/2(Enthalpy of Reheater Feedwater)
  [steam_flow_nc] -> MOISTURE SEPARATOR/3(Steam Flow Rate Nozzle Chest)
  [steam_bleed_hp] -> MOISTURE SEPARATOR/5(Steam Bleed Flow HP Turbine)
  CONDENSER/3(Condensate Flow Rate) -> Scope29/1, [flow_co_fwh1]
  FEEDWATER HEATER 2 - HIGH-PRESSURE/2(Flow to Feedwater Heater 1) -> Scope27/1, [flow_fwh2_fwh1], Display41/1
  [steam_flow_nc] -> HIGH PRESSURE TURBINE/1(Steam Flow Rate Nozzle Chest)
  [H_hp] -> MOISTURE SEPARATOR/6(Steam Enthalpy HP Turbine)
  HIGH PRESSURE TURBINE/2(Steam Bleed Flow HP Turbine) -> Scope13/1, [steam_bleed_hp], Display28/1
  [flow_ms_rh] -> REHEATER/2(Flow from Moisture Seperator Reheater)
  HIGH PRESSURE TURBINE/3(Steam Enthalpy HP Turbine) -> Scope15/1, [H_hp], Display27/1
  [steam_flow_reheat] -> REHEATER/1(Steam Flow Rate Secondary Valve)
  [steam_flow_nc] -> FEEDWATER HEATER 2 - HIGH-PRESSURE/7(Steam Flow Rate Nozzle Chest)
  [T_steam_OTSG] -> REHEATER/3(Steam Temperature)
  FEEDWATER HEATER 2 - HIGH-PRESSURE/1(Enthalpy of Feedwater Heater 2) -> Scope26/1, Display40/1
  CONDENSER/2(Pressure of Condenser) -> Scope1/1, Display44/1
  [H_co] -> FEEDWATER HEATER 1 - LOW-PRESSURE/4(Condenser Enthalpy)
  [steam_flow_lp] -> CONDENSER/1(Steam Flow Rate LP Turbine)
  FEEDWATER HEATER 1 - LOW-PRESSURE/1(Enthalpy of fluid from Feedwater Heater) -> Scope19/1, [H_fwh1], Display38/1
  [H_rh] -> LOW PRESSURE TURBINE/2(Steam Enthalpy Reheater)
  [steam_bleed_hp] -> FEEDWATER HEATER 2 - HIGH-PRESSURE/1(Steam Bleed Flow HP Turbine)
  FEEDWATER HEATER 2 - HIGH-PRESSURE/4(Temperature of Feedwater) -> Out Bus Element/1, Display46/1, Scope8/1
  [steam_flow_hp] -> MOISTURE SEPARATOR/4(Steam Flow Rate HP Turbine)
  CONDENSER/1(Enthalpy of Condenser) -> Scope2/1, [H_co], Display43/1
  REHEATER/4(Steam Enthalpy Reheater) -> Scope18/1, [H_rh], Display35/1
  [flow_co_fwh1] -> FEEDWATER HEATER 1 - LOW-PRESSURE/1(Steam Flow Rate LP Turbine)
  In Bus Element/1 -> [T_steam_OTSG]
  In Bus Element1/1 -> [P_steam_OTSG]
  In Bus Element2/1 -> [steam_flow_OTSG]
  Temperature of Cooling Water Input/1 -> CONDENSER/4(Temperature Cooling Water)
  NOZZLE CHEST/2(Enthalpy of Reheater Feedwater) -> Scope7/1, [H_rh_nc], Display7/1
  HIGH PRESSURE TURBINE/1(Steam Flow Rate HP Turbine) -> Scope12/1, [steam_flow_hp], Display29/1
  REHEATER/1(Flow to LP Turbine) -> Scope14/1, [flow_rh_lpt], Display32/1
  [flow_fwh2_OTSG] -> Out Bus Element1/1
  [T_steam_OTSG] -> Scope31/1, Steam Enthalpy/1
  Flow of Cooling Water Input/1 -> CONDENSER/3(Flow Rate Cooling Water)

== system MSBR_Plant/Nuclear Steam Supply System (NSSS) ==
  In Bus Element : Inport  PortName=Feedwater
  Coolant Salt Pumps : Subsystem
  MSBR : Subsystem
  Once-Through Steam Generator (OTSG) : Subsystem
  Primary Heat Exchanger Loops (Blanket and Fuel Salt HXs) : Subsystem
  Primary Pumps (Blanket and Fuel Salt) : Subsystem
  Out Bus Element : Outport  PortName=NSSS Steam
  wires:
  MSBR/1(Fuel Core Outlet Temp) -> Primary Heat Exchanger Loops (Blanket and Fuel Salt HXs)/3(Fuel Salt Temp HX Inlet)
  Once-Through Steam Generator (OTSG)/2(Coolant Salt OTSG Outlet) -> Primary Heat Exchanger Loops (Blanket and Fuel Salt HXs)/6(Coolant Salt Temp HX Inlet)
  MSBR/2(Blanket Core Outlet Temp) -> Primary Heat Exchanger Loops (Blanket and Fuel Salt HXs)/4(Blanket Salt Temp HX Inlet)
  Primary Pumps (Blanket and Fuel Salt)/2(Blanket Pumps) -> Primary Heat Exchanger Loops (Blanket and Fuel Salt HXs)/2(Blanket Salt Pump Input)
  Primary Pumps (Blanket and Fuel Salt)/1(Fuel Pumps) -> Primary Heat Exchanger Loops (Blanket and Fuel Salt HXs)/1(Fuel Salt Pump Input)
  Coolant Salt Pumps/1(Coolant Pumps) -> Primary Heat Exchanger Loops (Blanket and Fuel Salt HXs)/5(Coolant Salt Pump Input)
  Primary Heat Exchanger Loops (Blanket and Fuel Salt HXs)/1(Fuel & Blanket Salt Outlet) -> MSBR/1(Core Inlet)
  Primary Heat Exchanger Loops (Blanket and Fuel Salt HXs)/2(Coolant Salt Outlet) -> Once-Through Steam Generator (OTSG)/2(Coolant Salt Inlet)
  Once-Through Steam Generator (OTSG)/1(NSSS Output) -> Out Bus Element/1
  In Bus Element/1 -> Once-Through Steam Generator (OTSG)/1(Feedwater)

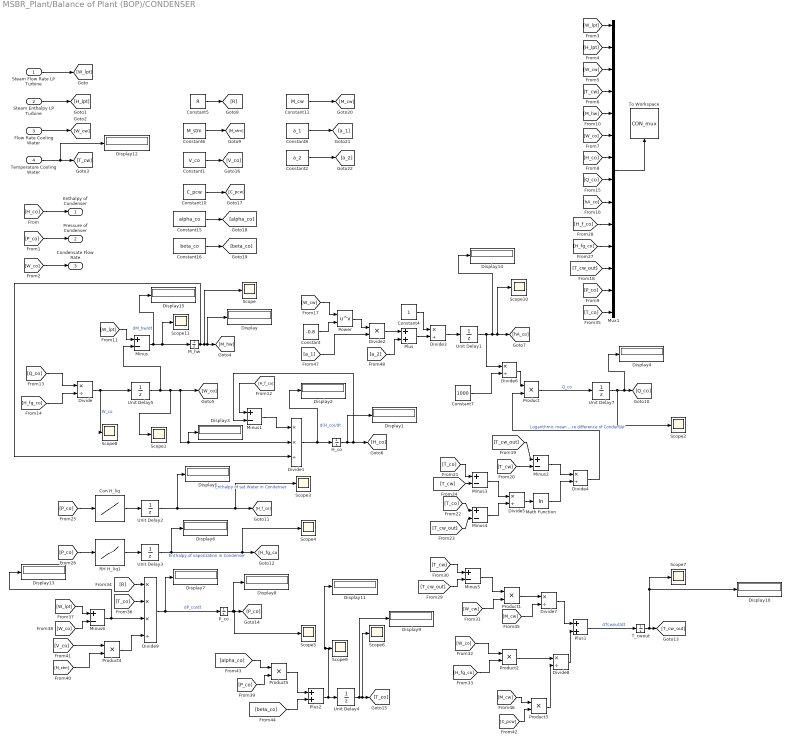
== system MSBR_Plant/Balance of Plant (BOP)/CONDENSER ==
  Steam Flow Rate LP Turbine : Inport
  Steam Enthalpy LP Turbine : Inport  Port=2
  Flow Rate Cooling Water : Inport  Port=3
  Temperature Cooling Water : Inport  Port=4
  Con H_liq : Lookup_n-D  NumberOfTableDimensions=1  BreakpointsForDimension1=P_con_table  Table=H_con_table  InternalRulePriority=Speed  RndMeth=Simplest  InputSameDT=on
  Constant : Constant  Value=-0.8
  Constant1 : Constant  Value=V_co
  Constant10 : Constant  Value=C_pcw
  Constant11 : Constant  Value=M_cw
  Constant15 : Constant  Value=alpha_co
  Constant16 : Constant  Value=beta_co
  Constant2 : Constant  Value=a_2
  Constant4 : Constant
  Constant5 : Constant  Value=R
  Constant6 : Constant  Value=M_stm
  Constant7 : Constant  Value=1000
  Constant8 : Constant  Value=a_1
  Display{,1..15} (16 alike) : Display
  Divide{,3..8} (7 alike) : Product  Inputs=*/
  Divide1 : Product  Inputs=**/
  Divide2 : Product  Inputs=**
  Divide9 : Product  Inputs=***/
  H_co : Integrator  InitialCondition=H_co0
  M_hw : Integrator  InitialCondition=M_hw0
  Math Function : Math  Operator=log  SaturateOnIntegerOverflow=on
  Minus{,1..6} (7 alike) : Sum  Inputs=+-
  Mux1 : Mux  Inputs=14
  P_co : Integrator  InitialCondition=P_co0
  Plus : Sum
  Plus1 : Sum
  Plus2 : Sum
  Power : Math  Operator=pow  SaturateOnIntegerOverflow=on
  Product{,1..5} (6 alike) : Product
  RH H_liq1 : Lookup_n-D  NumberOfTableDimensions=1  BreakpointsForDimension1=P_con_table  Table=H_convap_table  InternalRulePriority=Speed  RndMeth=Simplest  InputSameDT=on
  Scope{,1..11} (12 alike) : Scope
  T_cwout : Integrator  InitialCondition=T_cwout0
  To Workspace : ToWorkspace  VariableName=CON_mux  SaveFormat=Timeseries  SampleTime=0.1
      settings: Save2DSignal=2-D array (concatenate along first dimension)
  Unit Delay1 : UnitDelay  InitialCondition=hA_co0  SampleTime=-1  HasFrameUpgradeWarning=on
  Unit Delay2 : UnitDelay  InitialCondition=H_f_co0  SampleTime=-1  HasFrameUpgradeWarning=on
  Unit Delay3 : UnitDelay  InitialCondition=H_fg_co0  SampleTime=-1  HasFrameUpgradeWarning=on
  Unit Delay4 : UnitDelay  InitialCondition=T_co0  SampleTime=-1  HasFrameUpgradeWarning=on
  Unit Delay5 : UnitDelay  InitialCondition=W_co0  SampleTime=-1  HasFrameUpgradeWarning=on
  Unit Delay7 : UnitDelay  InitialCondition=Q_co0  SampleTime=-1  HasFrameUpgradeWarning=on
  Enthalpy of Condenser : Outport  VectorParamsAs1DForOutWhenUnconnected=off
  Pressure of Condenser : Outport  Port=2  VectorParamsAs1DForOutWhenUnconnected=off
  Condensate Flow Rate : Outport  Port=3  VectorParamsAs1DForOutWhenUnconnected=off
  wires:
  Steam Flow Rate LP Turbine/1 -> [W_lpt]
  Steam Enthalpy LP Turbine/1 -> [H_lpt]
  Flow Rate Cooling Water/1 -> [W_cw]
  Temperature Cooling Water/1 -> Display12/1, [T_cw]
  H_co/1 -> Display1/1, Minus1/2, [H_co]
  Unit Delay7/1 -> Scope2/1, Display4/1, [Q_co]
  Unit Delay1/1 -> Divide6/1, Display14/1, Scope10/1, [hA_co]
  Unit Delay2/1 -> Display5/1, Scope3/1, [H_f_co]  "Enthalpy of sat Water in Condenser"
  Unit Delay3/1 -> Display6/1, Scope4/1, [H_fg_co]  "Enthalpy of vaporization in Condenser"
  T_cwout/1 -> Display10/1, Scope7/1, [T_cw_out]
  P_co/1 -> Display8/1, Scope5/1, [P_co]
  Unit Delay4/1 -> Display9/1, Scope6/1, [T_co]
  Con H_liq/1 -> Unit Delay2/1
  RH H_liq1/1 -> Unit Delay3/1
  [H_co] -> Enthalpy of Condenser/1
  [P_co] -> Pressure of Condenser/1
  [W_co] -> Condensate Flow Rate/1
  [W_lpt] -> Mux1/1
  [H_lpt] -> Mux1/2
  [W_cw] -> Mux1/3
  [T_cw] -> Mux1/4
  [W_co] -> Mux1/6
  [H_co] -> Mux1/7
  [P_co] -> Mux1/13
  [M_hw] -> Mux1/5
  Minus/1 -> Display15/1, Scope11/1, M_hw/1  "dM_hw/dt"
  [W_lpt] -> Minus/1
  Unit Delay5/1 -> Minus/2, Scope1/1, Display3/1, Divide1/2, [W_co]
  Divide/1 -> Scope8/1, Unit Delay5/1  "W_co"
  [Q_co] -> Divide/1
  [H_fg_co] -> Divide/2
  [Q_co] -> Mux1/8
  Divide1/1 -> Display2/1, H_co/1  "d(H_co)/dt"
  Minus1/1 -> Divide1/1
  [H_f_co] -> Minus1/1
  [hA_co] -> Mux1/9
  [W_cw] -> Power/1
  Constant/1 -> Power/2
  [a_1] -> Divide2/2
  Power/1 -> Divide2/1
  Divide2/1 -> Plus/1
  Divide3/1 -> Unit Delay1/1
  Plus/1 -> Divide3/2
  Constant4/1 -> Divide3/1
  [T_cw_out] -> Mux1/12
  [T_cw_out] -> Minus2/1
  [T_cw] -> Minus2/2
  Minus2/1 -> Divide4/1
  Math Function/1 -> Divide4/2
  Divide5/1 -> Math Function/1
  Minus4/1 -> Divide5/2
  Minus3/1 -> Divide5/1
  [T_co] -> Minus4/1
  [T_co] -> Minus3/1
  [T_cw_out] -> Minus4/2
  [T_cw] -> Minus3/2
  Divide4/1 -> Product/2  "Logarithmic mean temperature difference of Condenser"
  Product/1 -> Unit Delay7/1  "Q_co"
  [P_co] -> Con H_liq/1
  [P_co] -> RH H_liq1/1
  Constant7/1 -> Divide6/2
  Divide6/1 -> Product/1
  [H_fg_co] -> Mux1/11
  [H_f_co] -> Mux1/10
  [T_cw] -> Minus5/1
  [T_cw_out] -> Minus5/2
  [W_cw] -> Product1/2
  Minus5/1 -> Product1/1
  Product1/1 -> Divide7/1
  [M_cw] -> Divide7/2
  Divide7/1 -> Plus1/1
  [W_co] -> Product2/1
  [H_fg_co] -> Product2/2
  Product2/1 -> Divide8/1
  [M_cw] -> Product3/1
  Product3/1 -> Divide8/2
  Divide8/1 -> Plus1/2
  Plus1/1 -> T_cwout/1  "dTcwout/dt"
  Constant5/1 -> [R]
  Constant6/1 -> [M_stm]
  [R] -> Divide9/1
  Minus6/1 -> Display13/1, Divide9/3
  [T_co] -> Mux1/14
  [T_co] -> Divide9/2
  [W_lpt] -> Minus6/1
  [W_co] -> Minus6/2
  Product4/1 -> Divide9/4
  [M_stm] -> Product4/2
  [V_co] -> Product4/1
  Divide9/1 -> P_co/1, Display7/1  "dP_co/dt"
  [alpha_co] -> Product5/1
  [P_co] -> Product5/2
  Product5/1 -> Plus2/1
  [beta_co] -> Plus2/2
  Plus2/1 -> Display11/1, Scope9/1, Unit Delay4/1
  Mux1/1 -> To Workspace/1
  Constant1/1 -> [V_co]
  Constant10/1 -> [C_pcw]
  [C_pcw] -> Product3/2
  Constant16/1 -> [beta_co]
  Constant15/1 -> [alpha_co]
  Constant11/1 -> [M_cw]
  Constant8/1 -> [a_1]
  Constant2/1 -> [a_2]
  [a_2] -> Plus/2
  M_hw/1 -> Scope/1, Display/1, [M_hw], Divide1/3

== system MSBR_Plant/Balance of Plant (BOP)/FEEDWATER HEATER 1 - LOW-PRESSURE ==
  Steam Flow Rate LP Turbine : Inport
  Steam Bleed Flow Rate LP Turbine : Inport  Port=2
  Flow from Feedwater Heater 2 : Inport  Port=3
  Condenser Enthalpy : Inport  Port=4
  Constant : Constant  Value=tau_fwh1
  Constant1 : Constant  Value=h_fwh1
  Divide : Product  Inputs=*/
  Divide1 : Product  Inputs=*/
  H_fwh1 : Integrator  InitialCondition=H_fwh10
  Minus : Sum  Inputs=+-
  Mux1 : Mux  Inputs=7
  Plus : Sum
  Product : Product
  Product1 : Product
  Sum : Sum  Inputs=++|
  Sum1 : Sum  Inputs=+++
  To Workspace : ToWorkspace  VariableName=FWH1_mux  SaveFormat=Timeseries  SampleTime=-1
      settings: Save2DSignal=2-D array (concatenate along first dimension)
  Unit Delay1 : UnitDelay  InitialCondition=W_fw  SampleTime=-1  HasFrameUpgradeWarning=on
  Unit Delay7 : UnitDelay  InitialCondition=Q_fwh10  SampleTime=-1  HasFrameUpgradeWarning=on
  Enthalpy of fluid from Feedwater Heater : Outport  VectorParamsAs1DForOutWhenUnconnected=off
  Feedwater Flow Rate : Outport  Port=2  VectorParamsAs1DForOutWhenUnconnected=off
  wires:
  Steam Flow Rate LP Turbine/1 -> [W_lpt]
  Steam Bleed Flow Rate LP Turbine/1 -> [W_blp]
  Flow from Feedwater Heater 2/1 -> [W_hp_lp]
  Condenser Enthalpy/1 -> [H_co]
  H_fwh1/1 -> [H_fwh1]
  Unit Delay7/1 -> [Q_fwh1]
  Unit Delay1/1 -> [W_fw]
  Mux1/1 -> To Workspace/1
  [W_fw] -> Feedwater Flow Rate/1
  [H_fwh1] -> Enthalpy of fluid from Feedwater Heater/1
  [W_lpt] -> Mux1/1
  [W_blp] -> Mux1/2
  [W_hp_lp] -> Mux1/3
  [H_co] -> Mux1/4
  [H_fwh1] -> Mux1/5
  [Q_fwh1] -> Mux1/6
  [W_fw] -> Mux1/7
  Constant/1 -> [tau_fwh1]
  Constant1/1 -> [h_fwh1]
  [Q_fwh1] -> Divide/1
  [tau_fwh1] -> Product/1
  [W_fw] -> Product/2
  Product/1 -> Divide/2
  Divide/1 -> Plus/1
  [H_co] -> Minus/1
  [H_fwh1] -> Minus/2
  Minus/1 -> Divide1/1
  [tau_fwh1] -> Divide1/2
  Divide1/1 -> Plus/2
  Plus/1 -> H_fwh1/1  "dH_fwh1/dt"
  [W_blp] -> Sum/1
  [W_hp_lp] -> Sum/2
  Sum/1 -> Product1/2
  [h_fwh1] -> Product1/1
  Product1/1 -> Unit Delay7/1
  [W_hp_lp] -> Sum1/3
  [W_blp] -> Sum1/2
  [W_lpt] -> Sum1/1
  Sum1/1 -> Unit Delay1/1

== system MSBR_Plant/Balance of Plant (BOP)/FEEDWATER HEATER 2 - HIGH-PRESSURE ==
  Steam Bleed Flow HP Turbine : Inport
  Flow from Moisture Seperator : Inport  Port=2
  Flow from Reheater : Inport  Port=3
  "Flow from Moisture Seperator to Reheater " : Inport  Port=4
  Flow from Feedwater Heater 1 : Inport  Port=5
  Enthalpy of Feedwater Heater 1 : Inport  Port=6
  Steam Flow Rate Nozzle Chest : Inport  Port=7
  Constant : Constant  Value=tau_fwh2
  Constant1 : Constant  Value=h_fwh2
  Constant2 : Constant  Value=tau_rh2
  Constant3 : Constant  Value=Cp_fw
  Divide{,1..2,4..5} (5 alike) : Product  Inputs=*/
  Divide3 : Product  Inputs=**
  H_fwh : Integrator  InitialCondition=H_fwh20
  Minus : Sum  Inputs=+-
  Minus1 : Sum  Inputs=+++-
  Minus2 : Sum
  Minus3 : Sum  Inputs=+-
  Mux1 : Mux  Inputs=11
  Product : Product
  Product1 : Product
  Sum : Sum  Inputs=|++
  Sum1 : Sum  Inputs=+++
  T_fw : Integrator  InitialCondition=T_fw
  To Workspace : ToWorkspace  VariableName=FWH2_mux  SaveFormat=Timeseries  SampleTime=-1
      settings: Save2DSignal=2-D array (concatenate along first dimension)
  Unit Delay7 : UnitDelay  InitialCondition=Q_fwh20  SampleTime=-1  HasFrameUpgradeWarning=on
  W_hp_lp : Integrator  InitialCondition=w_fwh
  Enthalpy of Feedwater Heater 2 : Outport  VectorParamsAs1DForOutWhenUnconnected=off
  Flow to Feedwater Heater 1 : Outport  Port=2  VectorParamsAs1DForOutWhenUnconnected=off
  Feedwater Flow Rate : Outport  Port=3  VectorParamsAs1DForOutWhenUnconnected=off
  Temperature of Feedwater : Outport  Port=4  VectorParamsAs1DForOutWhenUnconnected=off
  wires:
  Steam Bleed Flow HP Turbine/1 -> [W_bhp]
  Flow from Moisture Seperator/1 -> [W_liq]
  Flow from Reheater/1 -> [W_vrh]
  "Flow from Moisture Seperator to Reheater "/1 -> [W_ms]
  H_fwh/1 -> [H_fwh2]
  Unit Delay7/1 -> [Q_fwh2]
  Flow from Feedwater Heater 1/1 -> [W_fw], Feedwater Flow Rate/1
  Enthalpy of Feedwater Heater 1/1 -> [H_fwh1]
  Steam Flow Rate Nozzle Chest/1 -> [W_nc]
  W_hp_lp/1 -> [W_hp_lp]
  T_fw/1 -> [T_fw]
  [T_fw] -> Temperature of Feedwater/1
  [W_hp_lp] -> Flow to Feedwater Heater 1/1
  [H_fwh2] -> Enthalpy of Feedwater Heater 2/1
  [W_bhp] -> Mux1/1
  [W_liq] -> Mux1/2
  [W_vrh] -> Mux1/3
  [W_ms] -> Mux1/4
  [W_fw] -> Mux1/5
  [H_fwh1] -> Mux1/6
  [W_nc] -> Mux1/7
  [Q_fwh2] -> Mux1/9
  [W_hp_lp] -> Mux1/10
  [T_fw] -> Mux1/11
  [H_fwh2] -> Mux1/8
  Mux1/1 -> To Workspace/1
  Constant/1 -> [tau_fwh2]
  Constant1/1 -> [h_fwh2]
  Constant2/1 -> [tau_rh2]
  [tau_fwh2] -> Product/2
  [W_fw] -> Product/1
  Product/1 -> Divide/2
  [Q_fwh2] -> Divide/1
  Divide/1 -> Sum/1, Minus2/1
  Sum/1 -> H_fwh/1  "dH_fw/dt"
  Divide1/1 -> Sum/2
  Minus/1 -> Divide1/1
  [tau_fwh2] -> Divide1/2
  [H_fwh1] -> Minus/1
  [H_fwh2] -> Minus/2
  Product1/1 -> Unit Delay7/1  "Q_fwh2"
  [h_fwh2] -> Product1/1
  Sum1/1 -> Product1/2
  [W_bhp] -> Sum1/1
  [W_liq] -> Sum1/2
  [W_vrh] -> Sum1/3
  Minus1/1 -> Divide2/1
  Divide2/1 -> W_hp_lp/1  "dW_hp_lp/dt"
  [tau_rh2] -> Divide2/2
  [W_bhp] -> Minus1/1
  [W_liq] -> Minus1/2
  [W_vrh] -> Minus1/3
  [W_hp_lp] -> Minus1/4
  [H_fwh1] -> Minus3/1
  Constant3/1 -> [Cp_fw]
  Divide3/1 -> Minus3/2
  [Cp_fw] -> Divide3/1
  [T_fw] -> Divide3/2
  Minus3/1 -> Divide4/1
  Divide4/1 -> Minus2/2
  [tau_fwh2] -> Divide4/2
  Minus2/1 -> Divide5/1
  [Cp_fw] -> Divide5/2
  Divide5/1 -> T_fw/1  "dT_fw/dt"
